simulink model "PendoloSimulink"  (R2022b)
settings: Solver=FixedStepAuto  StartTime=0.0  StopTime=60  FixedStep=1/frameRate  MaxStep=1/frameRate  RelTol=1e-3
InitFcn:
  | StartCond
StopFcn:
  | % PlotResult
values from neighbouring files (symbols this model uses):
  g = 9.81    [StartCond.m]    (also in pendPlotFrame.m; pend_fn.m)
  K_p = 10    [StartCond.m]
  Kattr = 0.01    [StartCond.m]    (also in simScript.m = 0.1)
  Km = 0.7    [StartCond.m]    (also in simScript.m = 1)
  L = 2    [StartCond.m]    (also in simScript.m)
  Theta_Ref_max = deg2rad(30)    [StartCond.m]
  y0 = [deg2rad(degStart);0]    [StartCond.m]    (also in simScript.m = [deg2rad(degStart),0])
libraries: simulink x1
settings Model: Creator=alfy  LastModifiedBy=alfy
settings DataIOCC: SaveOutput=off  ReturnWorkspaceOutputs=off

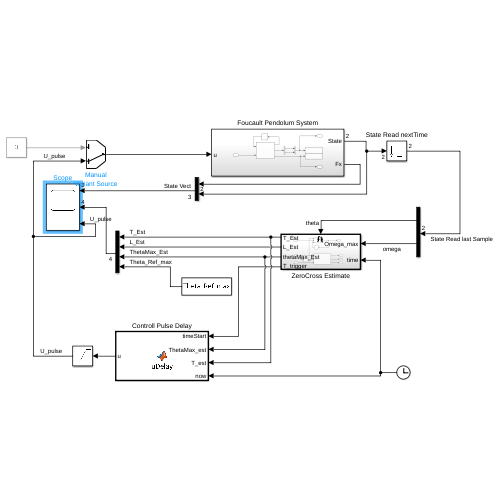
[thumbnail: Simulink's stored preview of the top-level diagram]
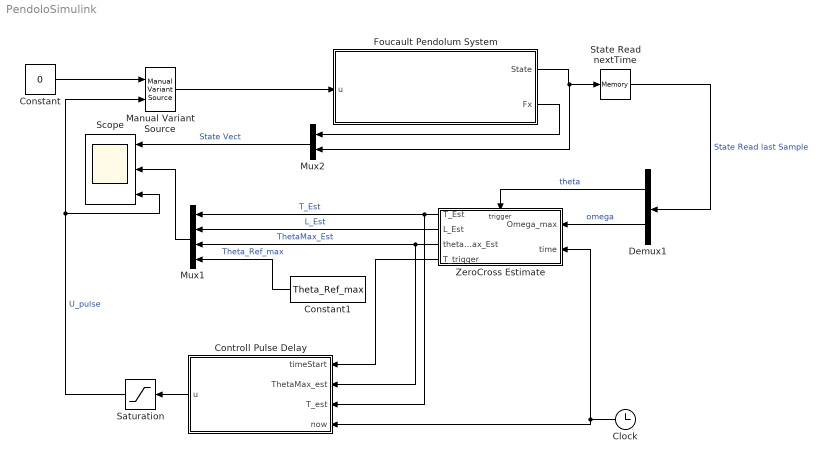
== system PendoloSimulink ==
  Clock : Clock
  Constant : Constant  Value=0
  Constant1 : Constant  Value=Theta_Ref_max
  Controll Pulse Delay : MATLAB Function  TreatAsAtomicUnit=on
  Demux1 : Demux  Outputs=2
  Foucault Pendolum System : Subsystem
  Manual Variant Source : simulink/Signal Routing/Manual Variant Source  NumChoices=2  LabelModeActiveChoice=V_2
  Mux1 : Mux
  Mux2 : Mux  Inputs=2
  Saturation : Saturate  UpperLimit=1  LowerLimit=0
  Scope : Scope  NumInputPorts=3
  State Read nextTime : Memory  InheritSampleTime=on
  ZeroCross Estimate : Subsystem  TreatAsAtomicUnit=on
  wires:
  ZeroCross Estimate/1(T_Est) -> Mux1/1, Controll Pulse Delay/3(T_est)  "T_Est"
  ZeroCross Estimate/2(L_Est) -> Mux1/2  "L_Est"
  ZeroCross Estimate/3(thetaMax_Est) -> Mux1/3, Controll Pulse Delay/2(ThetaMax_est)  "ThetaMax_Est"
  Mux1/1 -> Scope/2
  ZeroCross Estimate/4(T_trigger) -> Controll Pulse Delay/1(timeStart)
  Clock/1 -> ZeroCross Estimate/2(time), Controll Pulse Delay/4(now)
  Constant/1 -> Manual Variant Source/1
  Controll Pulse Delay/1(u) -> Saturation/1
  State Read nextTime/1 -> Demux1/1  "State Read last Sample"
  Demux1/1 -> ZeroCross Estimate/Trigger  "theta"
  Demux1/2 -> ZeroCross Estimate/1(Omega_max)  "omega"
  Manual Variant Source/1 -> Foucault Pendolum System/1(u)
  Foucault Pendolum System/1(State) -> Mux2/2, State Read nextTime/1
  Foucault Pendolum System/2(Fx) -> Mux2/1
  Mux2/1 -> Scope/1  "State Vect"
  Saturation/1 -> Manual Variant Source/2, Scope/3  "U_pulse"
  Constant1/1 -> Mux1/4  "Theta_Ref_max"

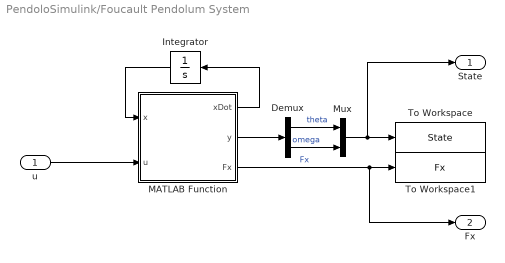
== system PendoloSimulink/Foucault Pendolum System ==
  u : Inport
  Demux : Demux  Outputs=2
  Integrator : Integrator  InitialCondition=y0
  MATLAB Function : MATLAB Function  TreatAsAtomicUnit=on
  Mux : Mux  Inputs=2
  To Workspace : ToWorkspace  VariableName=State  SaveFormat=Structure With Time  SampleTime=-1
      settings: Save2DSignal=2-D array (concatenate along first dimension)
  To Workspace1 : ToWorkspace  VariableName=Fx  SaveFormat=Structure With Time  SampleTime=-1
      settings: Save2DSignal=2-D array (concatenate along first dimension)
  State : Outport
  Fx : Outport  Port=2
  wires:
  MATLAB Function/1(xDot) -> Integrator/1
  u/1 -> MATLAB Function/2(u)
  Demux/2 -> Mux/2  "omega"
  MATLAB Function/2(y) -> Demux/1
  Integrator/1 -> MATLAB Function/1(x)
  Demux/1 -> Mux/1  "theta"
  MATLAB Function/3(Fx) -> Fx/1, To Workspace1/1  "Fx"
  Mux/1 -> State/1, To Workspace/1

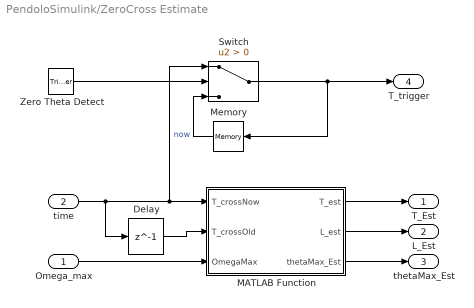
== system PendoloSimulink/ZeroCross Estimate ==
  Omega_max : Inport
  time : Inport  Port=2
  Zero Theta Detect : TriggerPort  TriggerType=either  VariantControl=(inherit)  ShowOutputPort=on
  Delay : Delay  DelayLength=1  InitialCondition=0
  MATLAB Function : MATLAB Function  TreatAsAtomicUnit=on
  Memory : Memory  InheritSampleTime=on
  Switch : Switch  Criteria=u2 > Threshold  SaturateOnIntegerOverflow=off  InputSameDT=off
  T_Est : Outport
  L_Est : Outport  Port=2
  thetaMax_Est : Outport  Port=3
  T_trigger : Outport  Port=4
  wires:
  Omega_max/1 -> MATLAB Function/3(OmegaMax)
  time/1 -> Delay/1, Switch/1, MATLAB Function/1(T_crossNow)  "now"
  Delay/1 -> MATLAB Function/2(T_crossOld)
  MATLAB Function/1(T_est) -> T_Est/1
  MATLAB Function/2(L_est) -> L_Est/1
  MATLAB Function/3(thetaMax_Est) -> thetaMax_Est/1
  Zero Theta Detect/1 -> Switch/2
  Switch/1 -> Memory/1, T_trigger/1
  Memory/1 -> Switch/3

== matlab function PendoloSimulink/ZeroCross Estimate/MATLAB Function ==
  data: T_crossNow input; T_est output; T_crossOld input; OmegaMax input; L_est output; g parameter; thetaMax_Est output; L parameter
function [T_est, L_est, thetaMax_Est] = fcn(T_crossNow, T_crossOld, OmegaMax, g, L)
if(T_crossOld == 0)
    % Aspetto di vedere almeno 2 passaggi
    [T_est, L_est, thetaMax_Est] = deal(0,0,0);
    return
end
T_est = (T_crossNow - T_crossOld) * 2; % Misuro mezzo periodo
L_est = (T_est/(2*pi))^2 * g;
VmaxNow = OmegaMax * L; % Nella realtà misuro V_max, quindi va bene
thetaMax_Est = acos(1 - VmaxNow^2/(2*g*L_est));
end

== matlab function PendoloSimulink/Foucault Pendolum System/MATLAB Function ==
  data: x input; xDot output; u input; y output; L parameter; Km parameter; Kattr parameter; g parameter; Fx output
function [xDot,y,Fx] = pendDinamic(x,u, L, Km, Kattr, g)
% x   = [theta, omega]

[theta, omega] = deal(x(1), x(2));

% Matrice dinamica interna non lineare nei parametri
F_state = [              omega;
           -g/L*sin(theta) - Kattr * omega];

% Matrice controllo non lineare nei coefficienti
Fm_x = -sign(theta)* Km * cos(theta)/(1 + abs(L*sin(theta)))^2;

B_state = [     0;
              Fm_x];

xDot= F_state + B_state * abs(u);
y = [theta; omega];
Fx = Fm_x * abs(u);
end

== matlab function PendoloSimulink/Controll Pulse Delay ==
  data: timeStart input; ThetaMax_est input; T_est input; u output; now input; K_p parameter; Theta_Ref_max parameter
function u = uDelay(timeStart, ThetaMax_est, T_est, now, K_p, Theta_Ref_max)

if now == 0 || timeStart == 0
    u=0;
    return
end

THalf = T_est/2;
err = Theta_Ref_max - ThetaMax_est;

% THalf*0.51 = Inizio discesa + eps
TStartCtrl = THalf*0.51;

% ThetaMax_est*0.45 = Fattore che estende la durata del controllo all'aumentare della velocità angolare => Sposto lo spegnimento più vicino all'origine
% THalf*0.7  = Avendo l'accelerazione magnetica, poco prima di superare l'asse, EMPIRICO
tSum = ThetaMax_est*0.5; % Trasforma una configurazione che non raggiunge l'obiettivo in una che riesce (minore forza magnetica necessaria), all'aumentare dell'obiettivo, deve diminuire
% Nel caso reale, se si riesce a detectare il passaggio in 0, spegnere a quel punto

TEndCtrl = THalf*0.7 + tSum;

if(((timeStart + TStartCtrl) <= now)  && (now <= (timeStart + TEndCtrl)))
    u = err * K_p;
else
    u = 0;
end
end
